simulink model "TADPOLE_Closed_Loop_NEWPLANT"  (R2024b)
settings: Solver=VariableStepAuto  StartTime=0.0  StopTime=19  RelTol=1e-3
InitFcn:
  | clear mex;
values from neighbouring files (symbols this model uses):
  timeDelta = 1/5000    (= 0.0002)    [TADPOLEControl.m]
  timeDeltaOUT = 1/1000    (= 0.001)    [TADPOLEControl.m]
  x0 = [0 0 0 0]    [TADPOLEControl.m]
settings Model: Creator=pplat  LastModifiedBy=pplat
settings DebuggingCC: AlgebraicLoopMsg=none

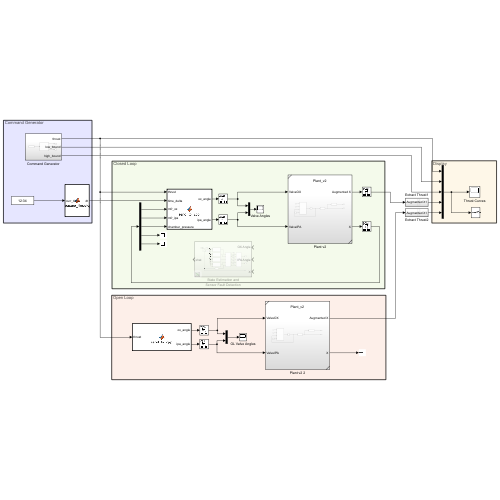
[thumbnail: Simulink's stored preview of the top-level diagram]
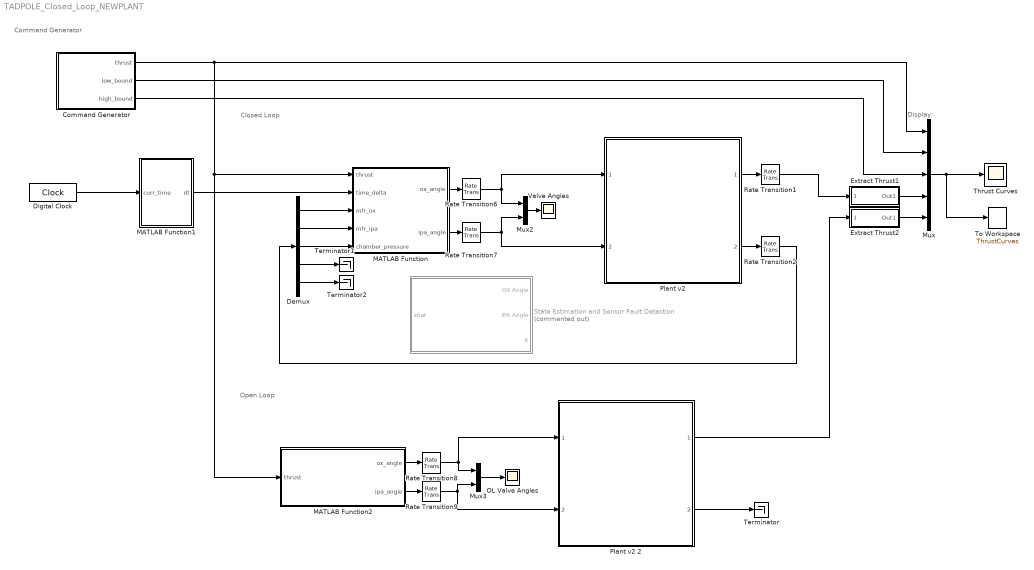
== system TADPOLE_Closed_Loop_NEWPLANT ==
  note: Display
  note: Open Loop
  note: Closed Loop
  note: Command Generator
  Command Generator : Subsystem
  Demux : Demux  Outputs=5
  Digital Clock : DigitalClock  SampleTime=timeDelta
  Extract Thrust1 : Subsystem
  Extract Thrust2 : Subsystem
  MATLAB Function : MATLAB Function  TreatAsAtomicUnit=on
  MATLAB Function1 : MATLAB Function  TreatAsAtomicUnit=on
  MATLAB Function2 : MATLAB Function  TreatAsAtomicUnit=on
  Mux : Mux  Inputs=5
  Mux2 : Mux  Inputs=2
  Mux3 : Mux  Inputs=2
  OL Valve Angles : Scope
  Plant v2 : Subsystem  ReferencedSubsystem=Plant_v2
  Plant v2 2 : Subsystem  ReferencedSubsystem=Plant_v2
  Rate Transition1 : RateTransition  OutPortSampleTime=timeDeltaOUT
  Rate Transition2 : RateTransition  OutPortSampleTime=timeDeltaOUT
  Rate Transition{6..9} (4 alike) : RateTransition  OutPortSampleTime=timeDeltaCMD
  State Estimation and Sensor Fault Detection : Subsystem  Commented=on
  Terminator : Terminator
  Terminator1 : Terminator
  Terminator2 : Terminator
  Thrust Curves : Scope
  To Workspace : ToWorkspace  VariableName=ThrustCurves  SaveFormat=Timeseries  SampleTime=-1
  Valve Angles : Scope
  wires:
  Mux/1 -> To Workspace/1, Thrust Curves/1
  MATLAB Function/2(ipa_angle) -> Rate Transition7/1
  MATLAB Function/1(ox_angle) -> Rate Transition6/1
  Mux2/1 -> Valve Angles/1
  Command Generator/1(thrust) -> Mux/1, MATLAB Function2/1(thrust), MATLAB Function/1(thrust)
  Command Generator/2(low_bound) -> Mux/2
  Command Generator/3(high_bound) -> Mux/3
  MATLAB Function1/1(dt) -> MATLAB Function/2(time_delta)
  Mux3/1 -> OL Valve Angles/1
  MATLAB Function2/1(ox_angle) -> Rate Transition8/1
  MATLAB Function2/2(ipa_angle) -> Rate Transition9/1
  Digital Clock/1 -> MATLAB Function1/1(curr_time)
  Rate Transition6/1 -> Mux2/1, Plant v2/1
  Rate Transition7/1 -> Plant v2/2, Mux2/2
  Rate Transition8/1 -> Plant v2 2/1, Mux3/1
  Rate Transition9/1 -> Plant v2 2/2, Mux3/2
  Extract Thrust1/1(Out1) -> Mux/4
  Extract Thrust2/1(Out1) -> Mux/5
  Plant v2/1 -> Rate Transition1/1
  Plant v2 2/1 -> Extract Thrust2/1(Augmented X)
  Plant v2 2/2 -> Terminator/1
  Rate Transition1/1 -> Extract Thrust1/1(Augmented X)
  Plant v2/2 -> Rate Transition2/1
  Demux/3 -> MATLAB Function/5(chamber_pressure)
  Demux/2 -> MATLAB Function/4(mfr_ipa)
  Demux/1 -> MATLAB Function/3(mfr_ox)
  Demux/4 -> Terminator1/1
  Demux/5 -> Terminator2/1
  Rate Transition2/1 -> Demux/1

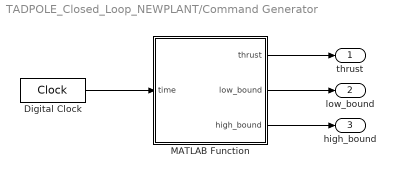
== system TADPOLE_Closed_Loop_NEWPLANT/Command Generator ==
  Digital Clock : DigitalClock  SampleTime=timeDelta
  MATLAB Function : MATLAB Function  TreatAsAtomicUnit=on
  thrust : Outport
  low_bound : Outport  Port=2
  high_bound : Outport  Port=3
  wires:
  MATLAB Function/1(thrust) -> thrust/1
  Digital Clock/1 -> MATLAB Function/1(time)
  MATLAB Function/2(low_bound) -> low_bound/1
  MATLAB Function/3(high_bound) -> high_bound/1

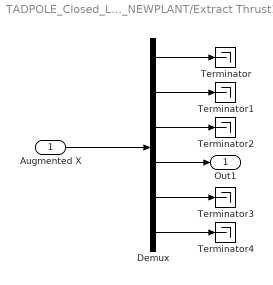
== system TADPOLE_Closed_Loop_NEWPLANT/Extract Thrust1 ==
  Augmented X : Inport
  Demux : Demux  Outputs=6
  Terminator{,1..4} (5 alike) : Terminator
  Out1 : Outport
  wires:
  Augmented X/1 -> Demux/1
  Demux/1 -> Terminator/1
  Demux/2 -> Terminator1/1
  Demux/3 -> Terminator2/1
  Demux/5 -> Terminator3/1
  Demux/6 -> Terminator4/1
  Demux/4 -> Out1/1

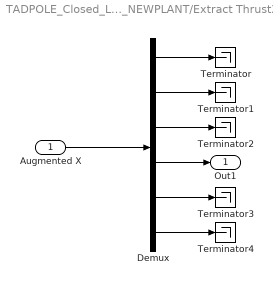
== system TADPOLE_Closed_Loop_NEWPLANT/Extract Thrust2 ==
  Augmented X : Inport
  Demux : Demux  Outputs=6
  Terminator{,1..4} (5 alike) : Terminator
  Out1 : Outport
  wires:
  Augmented X/1 -> Demux/1
  Demux/1 -> Terminator/1
  Demux/2 -> Terminator1/1
  Demux/3 -> Terminator2/1
  Demux/5 -> Terminator3/1
  Demux/6 -> Terminator4/1
  Demux/4 -> Out1/1

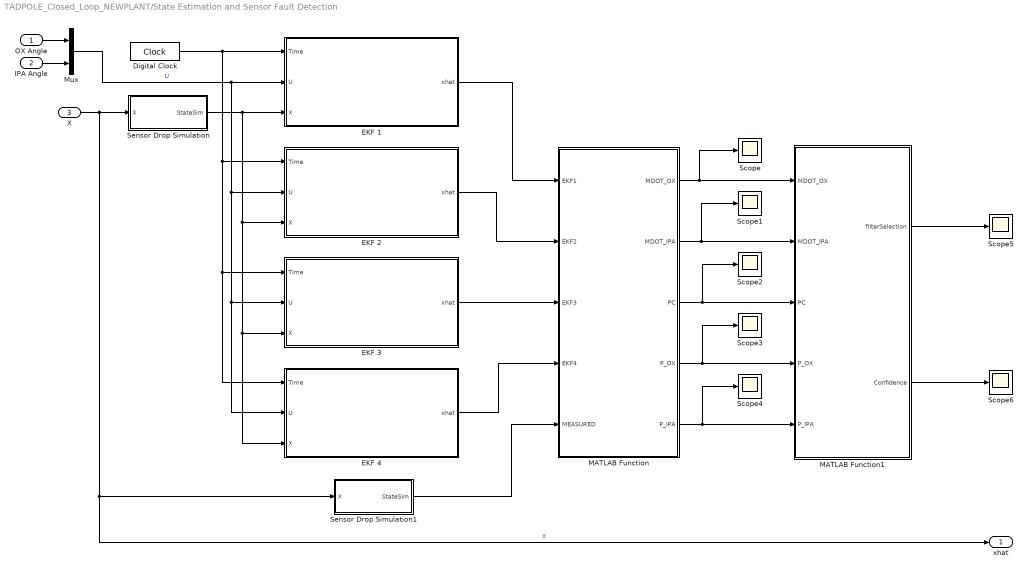
== system TADPOLE_Closed_Loop_NEWPLANT/State Estimation and Sensor Fault Detection ==
  OX Angle : Inport
  IPA Angle : Inport  Port=2
  X : Inport  Port=3
  Digital Clock : DigitalClock  SampleTime=timeDeltaOUT
  EKF 1 : Subsystem
  EKF 2 : Subsystem
  EKF 3 : Subsystem
  EKF 4 : Subsystem
  MATLAB Function : MATLAB Function  TreatAsAtomicUnit=on
  MATLAB Function1 : MATLAB Function  TreatAsAtomicUnit=on
  Mux : Mux  Inputs=2
  Scope{,1..6} (7 alike) : Scope
  Sensor Drop Simulation : Subsystem
  Sensor Drop Simulation1 : Subsystem
  xhat : Outport
  wires:
  IPA Angle/1 -> Mux/2
  OX Angle/1 -> Mux/1
  X/1 -> Sensor Drop Simulation/1(X), xhat/1, Sensor Drop Simulation1/1(X)  "X"
  Mux/1 -> EKF 3/2(U), EKF 4/2(U), EKF 2/2(U), EKF 1/2(U)  "U"
  Digital Clock/1 -> EKF 3/1(Time), EKF 4/1(Time), EKF 2/1(Time), EKF 1/1(Time)
  Sensor Drop Simulation/1(StateSim) -> EKF 2/3(X), EKF 3/3(X), EKF 4/3(X), EKF 1/3(X)
  EKF 1/1(xhat) -> MATLAB Function/1(EKF1)
  EKF 2/1(xhat) -> MATLAB Function/2(EKF2)
  EKF 3/1(xhat) -> MATLAB Function/3(EKF3)
  EKF 4/1(xhat) -> MATLAB Function/4(EKF4)
  Sensor Drop Simulation1/1(StateSim) -> MATLAB Function/5(MEASURED)
  MATLAB Function/5(P_IPA) -> MATLAB Function1/5(P_IPA), Scope4/1
  MATLAB Function/4(P_OX) -> MATLAB Function1/4(P_OX), Scope3/1
  MATLAB Function/3(PC) -> Scope2/1, MATLAB Function1/3(PC)
  MATLAB Function/2(MDOT_IPA) -> MATLAB Function1/2(MDOT_IPA), Scope1/1
  MATLAB Function/1(MDOT_OX) -> Scope/1, MATLAB Function1/1(MDOT_OX)
  MATLAB Function1/1(filterSelection) -> Scope5/1
  MATLAB Function1/2(Confidence) -> Scope6/1

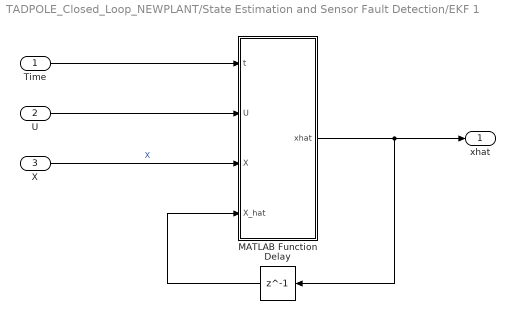
== system TADPOLE_Closed_Loop_NEWPLANT/State Estimation and Sensor Fault Detection/EKF 1 ==
  Time : Inport
  U : Inport  Port=2
  X : Inport  Port=3
  Delay : Delay  DelayLength=1  InitialCondition=x0.'
  MATLAB Function : MATLAB Function  TreatAsAtomicUnit=on
  xhat : Outport
  wires:
  Time/1 -> MATLAB Function/1(t)
  Delay/1 -> MATLAB Function/4(X_hat)
  MATLAB Function/1(xhat) -> xhat/1, Delay/1
  X/1 -> MATLAB Function/3(X)  "X"
  U/1 -> MATLAB Function/2(U)

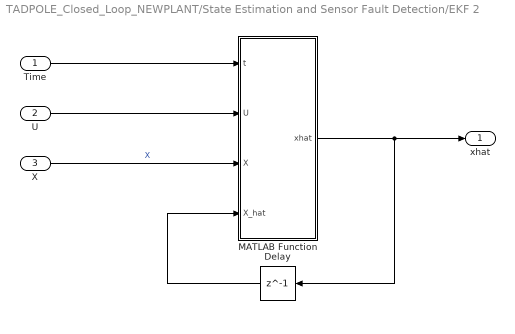
== system TADPOLE_Closed_Loop_NEWPLANT/State Estimation and Sensor Fault Detection/EKF 2 ==
  Time : Inport
  U : Inport  Port=2
  X : Inport  Port=3
  Delay : Delay  DelayLength=1  InitialCondition=x0.'
  MATLAB Function : MATLAB Function  TreatAsAtomicUnit=on
  xhat : Outport
  wires:
  Time/1 -> MATLAB Function/1(t)
  Delay/1 -> MATLAB Function/4(X_hat)
  MATLAB Function/1(xhat) -> xhat/1, Delay/1
  X/1 -> MATLAB Function/3(X)  "X"
  U/1 -> MATLAB Function/2(U)

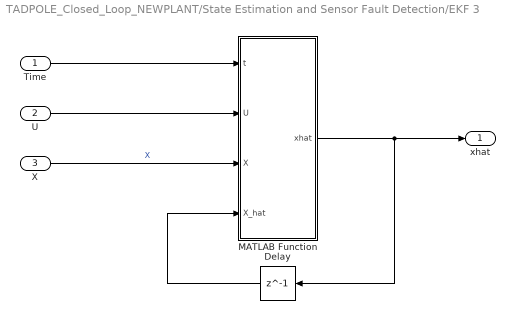
== system TADPOLE_Closed_Loop_NEWPLANT/State Estimation and Sensor Fault Detection/EKF 3 ==
  Time : Inport
  U : Inport  Port=2
  X : Inport  Port=3
  Delay : Delay  DelayLength=1  InitialCondition=x0.'
  MATLAB Function : MATLAB Function  TreatAsAtomicUnit=on
  xhat : Outport
  wires:
  Time/1 -> MATLAB Function/1(t)
  Delay/1 -> MATLAB Function/4(X_hat)
  MATLAB Function/1(xhat) -> xhat/1, Delay/1
  X/1 -> MATLAB Function/3(X)  "X"
  U/1 -> MATLAB Function/2(U)

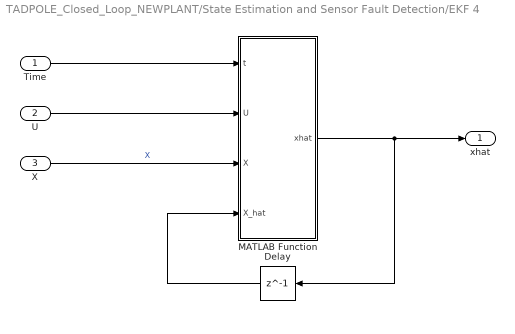
== system TADPOLE_Closed_Loop_NEWPLANT/State Estimation and Sensor Fault Detection/EKF 4 ==
  Time : Inport
  U : Inport  Port=2
  X : Inport  Port=3
  Delay : Delay  DelayLength=1  InitialCondition=x0.'
  MATLAB Function : MATLAB Function  TreatAsAtomicUnit=on
  xhat : Outport
  wires:
  Time/1 -> MATLAB Function/1(t)
  Delay/1 -> MATLAB Function/4(X_hat)
  MATLAB Function/1(xhat) -> xhat/1, Delay/1
  X/1 -> MATLAB Function/3(X)  "X"
  U/1 -> MATLAB Function/2(U)

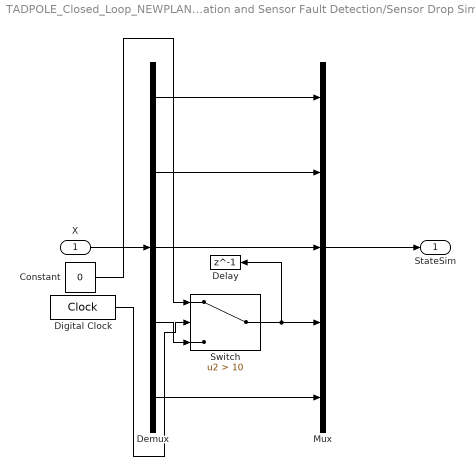
== system TADPOLE_Closed_Loop_NEWPLANT/State Estimation and Sensor Fault Detection/Sensor Drop Simulation ==
  X : Inport
  Constant : Constant  Value=0
  Delay : Delay  DelayLength=1
  Demux : Demux  Outputs=5
  Digital Clock : DigitalClock  SampleTime=timeDeltaOUT
  Mux : Mux  Inputs=5
  Switch : Switch  Criteria=u2 > Threshold  Threshold=10  SaturateOnIntegerOverflow=off  InputSameDT=off
  StateSim : Outport
  wires:
  X/1 -> Demux/1
  Mux/1 -> StateSim/1
  Demux/1 -> Mux/1
  Demux/2 -> Mux/2
  Demux/3 -> Mux/3
  Demux/5 -> Mux/5
  Digital Clock/1 -> Switch/2
  Switch/1 -> Delay/1, Mux/4
  Demux/4 -> Switch/3
  Constant/1 -> Switch/1

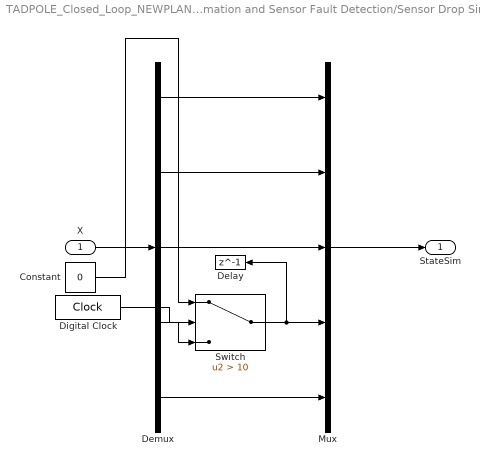
== system TADPOLE_Closed_Loop_NEWPLANT/State Estimation and Sensor Fault Detection/Sensor Drop Simulation1 ==
  X : Inport
  Constant : Constant  Value=0
  Delay : Delay  DelayLength=1
  Demux : Demux  Outputs=5
  Digital Clock : DigitalClock  SampleTime=timeDeltaOUT
  Mux : Mux  Inputs=5
  Switch : Switch  Criteria=u2 > Threshold  Threshold=10  SaturateOnIntegerOverflow=off  InputSameDT=off
  StateSim : Outport
  wires:
  X/1 -> Demux/1
  Mux/1 -> StateSim/1
  Demux/1 -> Mux/1
  Demux/2 -> Mux/2
  Demux/3 -> Mux/3
  Demux/5 -> Mux/5
  Digital Clock/1 -> Switch/2
  Switch/1 -> Delay/1, Mux/4
  Demux/4 -> Switch/3
  Constant/1 -> Switch/1

== matlab function TADPOLE_Closed_Loop_NEWPLANT/State Estimation and Sensor Fault Detection/MATLAB Function1 ==
  data: MDOT_OX input; filterSelection output; MDOT_IPA input; PC input; P_OX input; P_IPA input; Confidence output
function [filterSelection, Confidence] = Select(MDOT_OX, MDOT_IPA, PC, P_OX, P_IPA)
    
    [filterSelection, Confidence] = filterSelect(MDOT_OX, MDOT_IPA, PC, P_OX, P_IPA);
end

== matlab function TADPOLE_Closed_Loop_NEWPLANT/MATLAB Function ==
  data: thrust input; time_delta input; ox_angle output; ipa_angle output; mfr_ox input; mfr_ipa input; chamber_pressure input
function [ox_angle, ipa_angle] = send_to_cpp(thrust, time_delta, mfr_ox, mfr_ipa, chamber_pressure)
coder.extrinsic('closed_loop_valve_control_wrap');  % Declare MEX function as extrinsic
ox_angle = 0;
ipa_angle = 0;
[ox_angle, ipa_angle] = closed_loop_valve_control_wrap(thrust, time_delta, mfr_ox, mfr_ipa, chamber_pressure);

== matlab function TADPOLE_Closed_Loop_NEWPLANT/MATLAB Function1 ==
  data: dt output; curr_time input
function dt = measure_timestep(curr_time)
    persistent prev_time;
    if isempty(prev_time)
        prev_time = 0;
    end
    if curr_time < 0.3
        dt = 0;
    else
        dt = curr_time - prev_time;
    end
    prev_time = curr_time;
end

== matlab function TADPOLE_Closed_Loop_NEWPLANT/Command Generator/MATLAB Function ==
  data: time input; thrust output; low_bound output; high_bound output
function [thrust,low_bound,high_bound] = thrustCurveBounds(time)
thrust = CPLC(time);
t_past = CPLC(time - 0.5);
t_future = CPLC(time + 0.5);

high_bound = max([thrust, t_past, t_future]) + 0.05 * 550;
low_bound = min([thrust, t_past, t_future]) - 0.05 * 550;

end

== matlab function TADPOLE_Closed_Loop_NEWPLANT/MATLAB Function2 ==
  data: thrust input; ox_angle output; ipa_angle output
function [ox_angle, ipa_angle] = send_to_cpp(thrust)
coder.extrinsic('open_loop_valve_control_wrap');  % Declare MEX function as extrinsic
ox_angle = 0;
ipa_angle = 0;
[ox_angle, ipa_angle] = open_loop_valve_control_wrap(thrust);

== matlab function TADPOLE_Closed_Loop_NEWPLANT/State Estimation and Sensor Fault Detection/EKF 2/MATLAB Function ==
  data: t input; U input; X input; xhat output; X_hat input
function xhat = Estimate(t, U, X, X_hat)

    C = [0 0 0 1 0;
         0 0 0 0 1];
    
    xhat = EstimateState(X, X_hat, U, t, C);
end

== matlab function TADPOLE_Closed_Loop_NEWPLANT/State Estimation and Sensor Fault Detection/EKF 1/MATLAB Function ==
  data: t input; U input; X input; xhat output; X_hat input
function xhat = Estimate(t, U, X, X_hat)

    C = [0 0 1 0 0;
         0 0 0 1 0;
         0 0 0 0 1];
    
    xhat = EstimateState(X, X_hat, U, t, C);
end

== matlab function TADPOLE_Closed_Loop_NEWPLANT/State Estimation and Sensor Fault Detection/EKF 3/MATLAB Function ==
  data: t input; U input; X input; xhat output; X_hat input
function xhat = Estimate(t, U, X, X_hat)

    C = [0 0 1 0 0;
         0 0 0 0 1];
    
    xhat = EstimateState(X, X_hat, U, t, C);
end

== matlab function TADPOLE_Closed_Loop_NEWPLANT/State Estimation and Sensor Fault Detection/EKF 4/MATLAB Function ==
  data: t input; U input; X input; xhat output; X_hat input
function xhat = Estimate(t, U, X, X_hat)

    C = [0 0 1 0 0;
         0 0 0 1 0];
    
    xhat = EstimateState(X, X_hat, U, t, C);
end

== matlab function TADPOLE_Closed_Loop_NEWPLANT/State Estimation and Sensor Fault Detection/MATLAB Function ==
  data: EKF1 input; MDOT_OX output; EKF2 input; EKF3 input; EKF4 input; MEASURED input; MDOT_IPA output; PC output; P_OX output; P_IPA output
function [MDOT_OX, MDOT_IPA, PC, P_OX, P_IPA] = extractStates(EKF1, EKF2, EKF3, EKF4, MEASURED)

    MDOT_OX = [EKF1(1); EKF2(1); EKF3(1); EKF4(1); MEASURED(1)];
    MDOT_IPA = [EKF1(2); EKF2(2); EKF3(2); EKF4(2); MEASURED(2)];
    PC = [EKF1(3); EKF2(3); EKF3(3); EKF4(3); MEASURED(3)];
    P_OX = [EKF1(4); EKF2(4); EKF3(4); EKF4(4); MEASURED(4)];
    P_IPA = [EKF1(5); EKF2(5); EKF3(5); EKF4(5); MEASURED(5)];

end
